simulink model "test_MCU_RTI1202_20180630"  (R2017a)
settings: Solver=FixedStepDiscrete  StartTime=0.0  StopTime=Inf  FixedStep=0.05  RelTol=1e-3
PostLoadFcn:
  | , if any(exist('dsrtsu_mdlpostloadfcn', 'file') == [2, 3, 6]), try dsrtsu_mdlpostloadfcn('Execute', bdroot); catch fprintf('Error in PostLoadFcn (dsrtsu_mdlpostloadfcn) for model "%s":\n %s\n', bdroot, lasterr); end, end,
libraries: rti1202serlib x4
settings Model: DSRTSU_INTERNAL_RTI_VER=500  DSRTSU_INTERNAL_RTI_TYPE=rti1202  RTICANMMDATA=struct('GeneralSetupData',struct('modelroot',['L:\New folder\REC_Maroje\Demo1\RTI\Demos\Model\DS1202\Model'],'generalsettings',struct('filesettings',struct('destfolder',struct('Name','RTICANMM_FILES','Check',1),'buildfolder',struct('Name','.','Check',1),'AbsDestfolder',struct('Name',['L:\New folder\REC_Maroje\Demo1\RTI\Demos\Model\DS1202\Model\RTICANMM_FILES']),'AbsBuildfolder',struct('Name',['L:\New folder\REC_Maroje\Demo1\RTI\Demos\Model\DS1202\Model']))),'options',struct('addpaths',1,'rmpaths',1,'addtrcexclusion',logical(1),'cannavigator',struct('checkmonitoring',0),'show_usrtrc',0,'use_usrtrc',0),'advanced',struct('options',ones(1,100)),'MPSetup',{{}},'modelname','demo1202_serial_4','block','demo1202_serial_4'))  DSRTSU_INTERNAL_RTIFLEXRAYCONFIG=110  DSRTSU_INTERNAL_RTIFPGA=90  ExtModeTrigMode=oneshot  ExtModeArmWhenConnect=off  ExtModeAutoUpdateStatusClock=off  Creator=dSPACE GmbH  LastModifiedBy=kiritsuPC
settings DataIOCC: LimitDataPoints=on  SaveFormat=Array  SignalLoggingSaveFormat=ModelDataLogs
settings OptimizationCC: BlockReduction=off  ConditionallyExecuteInputs=off  OptimizeBlockIOStorage=off  BufferReuse=off  GlobalBufferReuse=off  ExpressionFolding=off  ExpressionDepthLimit=2147483647  LocalBlockOutputs=off  InitFltsAndDblsToZero=on  LifeSpan=inf
settings DebuggingCC: SaveWithParameterizedLinksMsg=none  UnderspecifiedInitializationDetection=Classic  MergeDetectMultiDrivingBlocksExec=none  SignalResolutionControl=TryResolveAllWithWarning  SolverPrmCheckMsg=warning  MultiTaskDSMMsg=warning  MultiTaskCondExecSysMsg=none  MultiTaskRateTransMsg=warning  TasksWithSamePriorityMsg=none  FcnCallInpInsideContextMsg=warning  AllowSymbolicDim=off  StateNameClashWarn=warning  SFUnexpectedBacktrackingDiag=warning  SFNoUnconditionalDefaultTransitionDiag=warning  SFExecutionAtInitializationDiag=none
settings HardwareCC: ProdBitPerPointer=32  ProdBitPerSizeT=32  ProdBitPerPtrDiffT=32  ProdLargestAtomicInteger=Integer  ProdEndianess=BigEndian  ProdWordSize=32  ProdHWDeviceType=Custom Processor->Custom  TargetIntDivRoundTo=Zero  TargetEndianess=BigEndian  TargetHWDeviceType=Custom Processor->Custom
settings ModelReferenceCC: PropagateSignalLabelsOutOfModel=off
settings SFSimCC: MATLABDynamicMemAlloc=off
settings RTWCC: SystemTargetFile=rti1202.tlc  MakeCommand=make_rti  TemplateMakefile=rti1202.tmf  Description=dSPACE DS1202 Hardware Platform  RTWVerbose=off
settings STFCustomTargetCC: ParMdlRefBuildCompliant=on  GRTInterface=off  SystemTargetFile=rti1202.tlc
settings GRTTargetCC: TargetLangStandard=C89/C90 (ANSI)  CompOptLevelCompliant=off  ConcurrentExecutionCompliant=off  CombineOutputUpdateFcns=off  MatFileLogging=off  CPPClassGenCompliant=off  UseToolchainInfoCompliant=off  ExtModeMexFile=noextcomm
settings ConfigComp: CovMetricSettings=dw  CovHtmlReporting=on  CovSaveCumulativeToWorkspaceVar=on  CovSaveSingleToWorkspaceVar=on  CovExternalEMLEnable=off

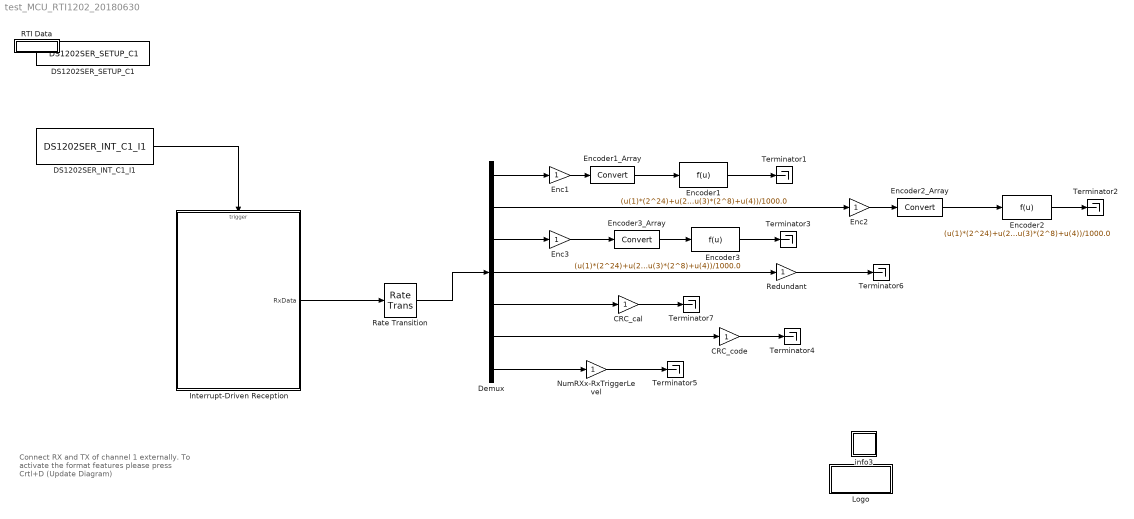
== system test_MCU_RTI1202_20180630 ==
  note: Connect RX and TX of channel 1 externally.
      | To activate the format features please
      | press Crtl+D (Update Diagram)
  CRC_cal : Gain  SaturateOnIntegerOverflow=on  OutDataTypeStr=Inherit: Same as input  ParamDataTypeStr=Inherit: Same as input
  CRC_code : Gain  SaturateOnIntegerOverflow=on  OutDataTypeStr=Inherit: Same as input  ParamDataTypeStr=Inherit: Same as input
  DS1202SER_INT_C1_I1 : rti1202serlib/DS1202SER_INT_C1_I1  Reserved1=[]  Reserved2=[]  Reserved3=[]  Reserved4=[]  DSProperties=struct('RTI',struct('IOBoardType',{{'DS1202','SER'}},'SlaveProcessor','NONE','Version',uint32(3),'BlockType',struct('isSLSource',uint8(1),'isSLSink',uint8(0),'isHWSource',uint8(0),'isHWSink',uint8(0),'isSetup',uint8(0),'isInline',uint8(1),'isNonInline',uint8(0),'isInterrupt',uint8(1),'isChannelwise',uint8(1)),'UnitType','GENSER','Identifier','SERINT','DialogType','ML','BlockSet','NONE','RelationId',struct('TH',struct('BlockId','HWINT'))))  RTIBlockInterface=struct('BlockDisplay',{{['DS1202 SER Interrupt\n Channel 1\nReceive Interrupt'],'center'}},'BlockName',struct('Token',{{'DS1202SER_INT_C','_I'}},'BlockParam',{{'ChannelNo','IntType'}}),'OutputPortsWidth',int32(1),'OutputPortsActive',1,'OutputPortsName',{{[' ']}},'IconTransparency','off','ParameterTunableNames',{{}},'InitLevel',3,'DialogFcn','guigenserserint','MaskDescription',['To make the interrupts of the UART serial interface available as trigger source.'],'FunctionCall',uint32(0),'Options',{{'SS_OPTION_FORCE_NONINLINED_FCNCALL','SS_OPTION_ASYNCHRONOUS_INTERRUPT'}})  RTIBlockParameters=struct('ThIntNo',{{'UART_EVENTS','OFF',[]}},'ThSubIntNo',{{0,'ON',[0 4]}},'ThSrcSgnName',{{['UART Ch1 RX SW FIFO interrupt'],'OFF',[]}},'TLCFileName',{{'rti_hwinterrupt','OFF',[]}},'BoardNo',{{1,'ON',[1 1]}},'ChannelNo',{{1,'ON',[1 2]}},'ChannelNumOf',{{2,'OFF',[]}},'ThBlk',{{['struct(''blkh'',''test_MCU_RTI1202_20180630/DS1202SER_INT_C1_I1'',''srcId'',''UART_EVENTS_CH1_INT0'',''srcSgnId'',''UART_EVENTS_CH1_INT0'',''intervalTmrBlockId'',[],''srcSgnName'',[''UART Ch1 RX SW FIFO interrupt''],''srcCpuId'','''',''isSrcCpu'',1,''isTargetCpu'',1,''srcOnMasterCpu'',1,''boardType'','''',''boardTypeNo'','''',''boardNo'',1,''intNo'',''UART_EVENTS'',''subIntNo'',0,''period'',0,''entryPoint'',''rti_UART_EVENTS_CH1_INT0'',''blockName'',''DS1202SER_INT_C1_I1'',''taskNameDisplayExt'','''',''taskType'',''HWINT'',''groupId'',''SERINT'',''hookFcn'',''NULL'',''isTimerTaskSrc'',0,''service'','''',''mpBlkId'','''',''taskPriorityPreConfig'',''none'',''taskPriority'',-1,''taskSortWeighting'',[],''taskSchedulingPolicy'',''FCFS'',''taskOvrPreConfig'',''none'',''taskOvrStrategy'',1,''taskOvrQueueSize'',1,''taskVisibility'',''on'',''taskGroupId'','''',''taskGroupDisplayOrder'',[],''serviceDynamicGen'',0,''disableCodeGen'',0,''boardBase'',''IOLIB_SPEC_INT_UART(1)'',''noBoardBase'','''')'],'OFF',[]}},'IntType',{{1,'ON',[1 4]}},'ReceiveIntLevelFifo',{{'13','OFF',[]}},'IntTypeMacro',{{'DSSER_TRIGGER_LEVEL_SUBINT_MASK','OFF',[]}},'FifoSizeDefault',{{64,'OFF',[]}})  RTISFcnParameters=struct('BoardNo','double','ChannelNo','double','ThIntNo','double','ThSubIntNo','double','ThBlk','struct','IntType','double','ReceiveIntLevelFifo','double','TLCFileName','char','IntTypeMacro','char')  RTIBlockParaDefault=struct('ThIntNo',1,'ThSubIntNo',0,'ThSrcSgnName',['RX SW FIFO interrupt'],'TLCFileName','rti_hwinterrupt','BoardNo',1,'ChannelNo',1,'ChannelNumOf',2,'ThBlk',['struct(''srcSgnId'', '''')'],'IntType',1,'ReceiveIntLevelFifo',1,'IntTypeMacro','DSSER_TRIGGER_LEVEL_SUBINT_MASK','FifoSizeDefault',64)
  DS1202SER_SETUP_C1 : rti1202serlib/DS1202SER_SETUP_C1  Reserved1=[]  Reserved2=[]  Reserved3=[]  Reserved4=[]  DSProperties=struct('RTI',struct('Version',uint32(2),'IOBoardType',{{'DS1202','SER'}},'SlaveProcessor','NONE','BlockType',struct('isSLSource',uint8(0),'isSLSink',uint8(0),'isHWSource',uint8(0),'isHWSink',uint8(0),'isSetup',uint8(1),'isInline',uint8(1),'isNonInline',uint8(0),'isInterrupt',uint8(0),'isChannelwise',uint8(1)),'UnitType','GENSER','Identifier','SETUP','DialogType','ML','BlockSet','NONE'))  RTIBlockInterface=struct('BlockName',struct('Token',{{'DS1202SER_SETUP_C'}},'BlockParam',{{'ChannelNo'}}),'BlockDisplay',{{['Serial Setup'],'center'}},'IconTransparency','off','ParameterTunableNames',{{}},'InitLevel',1,'DialogFcn','guigensersetup','MaskDescription',['To set the global specifications for the UART interface.'])  RTIBlockParameters=struct('ParityMode',{{1,'OFF',[1 5]}},'TransceiverMode',{{[3;1],'OFF',[]}},'QuartzFrequency',{{'160000000','OFF',[]}},'BoardNo',{{1,'ON',[1 1]}},'ChannelNo',{{1,'ON',[1 2]}},'ChannelNumOf',{{2,'OFF',[]}},'BaudRate',{{'115200','OFF',[]}},'DataBitsNumOf',{{4,'OFF',[1 4]}},'StopBitsNumOf',{{1,'OFF',[1 3]}},'ReceiveIntLevelUart',{{1,'OFF',[1 4]}},'AutoflowMode',{{0,'OFF',[]}},'FifoSize',{{'64','OFF',[]}},'ReceiveIntLevelFifo',{{0,'OFF',[]}},'FifoOverrunMode',{{1,'OFF',[]}},'FifoBlockSize',{{'0','OFF',[]}},'TermMode',{{1,'OFF',[]}},'TLCFileName',{{'rtigensersetup','OFF',[]}})  RTISFcnParameters=struct('BoardNo','double','ChannelNo','double','ChannelNumOf','double','BaudRate','double','DataBitsNumOf','double','StopBitsNumOf','double','ParityMode','double','TransceiverMode','double','ReceiveIntLevelUart','double','AutoflowMode','double','FifoSize','double','ReceiveIntLevelFifo','double','FifoBlockSize','double','TermMode','double','QuartzFrequency','double','TLCFileName','char')  RTIBlockParaDefault=struct('ParityMode',1,'TransceiverMode',[1;1],'QuartzFrequency',160000000,'BoardNo',1,'ChannelNo',1,'ChannelNumOf',2,'BaudRate',115200,'DataBitsNumOf',4,'StopBitsNumOf',1,'ReceiveIntLevelUart',4,'AutoflowMode',0,'FifoSize',64,'ReceiveIntLevelFifo',0,'FifoOverrunMode',1,'FifoBlockSize',0,'TermMode',1,'TLCFileName','rtigensersetup')
  Demux : Demux  Outputs=[4, 4, 4, 2, 1,1,2]
  Enc1 : Gain  SaturateOnIntegerOverflow=on  OutDataTypeStr=Inherit: Same as input  ParamDataTypeStr=Inherit: Same as input
  Enc2 : Gain  SaturateOnIntegerOverflow=on  OutDataTypeStr=Inherit: Same as input  ParamDataTypeStr=Inherit: Same as input
  Enc3 : Gain  SaturateOnIntegerOverflow=on  OutDataTypeStr=Inherit: Same as input  ParamDataTypeStr=Inherit: Same as input
  Encoder1 : Fcn  Expr=(u(1)*(2^24)+u(2)*(2^16)+u(3)*(2^8)+u(4))/1000.0
  "Encoder1_Array " : DataTypeConversion  SaturateOnIntegerOverflow=on  RndMeth=Zero
  Encoder2 : Fcn  Expr=(u(1)*(2^24)+u(2)*(2^16)+u(3)*(2^8)+u(4))/1000.0
  Encoder2_Array : DataTypeConversion  SaturateOnIntegerOverflow=on  RndMeth=Zero
  Encoder3 : Fcn  Expr=(u(1)*(2^24)+u(2)*(2^16)+u(3)*(2^8)+u(4))/1000.0
  "Encoder3_Array " : DataTypeConversion  SaturateOnIntegerOverflow=on  RndMeth=Zero
  Interrupt-Driven Reception : Subsystem  TreatAsAtomicUnit=on
  Logo : Subsystem  mask(dSPACE){EmptyParameter=[]}
      mask prompts: EmptyParameter "Mask Parameter 1:"
      settings: OpenFcn=;
      mask Display: image(imread('rti_mdl_dslogo.tif'));
  NumRXx-RxTriggerLevel : Gain  SaturateOnIntegerOverflow=on  OutDataTypeStr=Inherit: Same as input  ParamDataTypeStr=Inherit: Same as input
  RTI Data : Subsystem  Tag=struct('RTIDataServer',struct('RTIDataServerVs','2','RTIModelDescription','struct(''main'',''test_MCU_RTI1202_20180630'',''sub'','''',''isMp'',0)'))  LoadFcn="if exist('rtidc'), try,  rtidc('DataHostBlockClbLoad', gcbh); catch, disp(['Warning: ''LoadFcn'' for RTI Data block failed: ' lasterr]); end, end,"  mask(RTI_DATA_HOST){}
      mask help:
      | RTI Data Block.
      | This block is used by RTI to store internal model-dependent data.
      | Please keep this block on the root level of the model. Deleting this block will result in data loss.
      |
      | NEVER DELETE OR COPY THIS BLOCK!
      settings: CopyFcn="if exist('rtidc'), try,  rtidc('DataHostBlockClbCopy', gcbh); catch, disp(['Warning: ''CopyFcn'' for RTI Data block failed: ' lasterr]); end, end,"  DeleteFcn="if exist('rtidc'), try,  rtidc('DataHostBlockClbDelete', gcbh); catch, disp(['Warning: ''DeleteFcn'' for RTI Data block failed: ' lasterr]); end, end,"  ModelCloseFcn="if exist('rtidc'), try,  rtidc('DataHostBlockClbModelClose', gcbh); catch, disp(['Warning: ''ModelCloseFcn'' for RTI Data block failed: ' lasterr]); end, end,"  PreSaveFcn="if exist('rtidc'), try,  rtidc('DataHostBlockClbPreSave', gcbh); catch, disp(['Warning: ''PreSaveFcn'' for RTI Data block failed: ' lasterr]); end, end,"  PostSaveFcn="if exist('rtidc'), try,  rtidc('DataHostBlockClbPostSave', gcbh); catch, disp(['Warning: ''PostSaveFcn'' for RTI Data block failed: ' lasterr]); end, end,"  NameChangeFcn="if exist('rtidc'), try,  rtidc('DataHostBlockClbNameChange', gcbh); catch, disp(['Warning: ''NameChangeFcn'' for RTI Data block failed: ' lasterr]); end, end,"
      mask Help:
      | RTI Data Block.
      | This block is used by RTI to store internal model-dependent data.
      | Please keep this block on the root level of the model. Deleting this block will result in data loss.
      | 
      | NEVER DELETE OR COPY THIS BLOCK!
      mask Display:
      | text(0.5, 0.5, 'RTI Data', 'HorizontalAlignment', 'center');
      | plot([1 0]);
  Rate Transition : RateTransition  Integrity=off
  Redundant : Gain  SaturateOnIntegerOverflow=on  OutDataTypeStr=Inherit: Same as input  ParamDataTypeStr=Inherit: Same as input
  Terminator{1..7} (7 alike) : Terminator
  info3 : Subsystem
      settings: OpenFcn=web(fullfile(dspaceroot, 'demos', rtitype('processorboard'), 'rti', 'demo1xxx_serial_4.html'), '-browser');
      mask Display: disp('?')
  wires:
  DS1202SER_INT_C1_I1/1 -> Interrupt-Driven Reception/Trigger
  Interrupt-Driven Reception/1(RxData) -> Rate Transition/1
  Rate Transition/1 -> Demux/1
  NumRXx-RxTriggerLevel/1 -> Terminator5/1
  CRC_code/1 -> Terminator4/1
  Encoder3/1 -> Terminator3/1
  Encoder2/1 -> Terminator2/1
  Encoder1/1 -> Terminator1/1
  Redundant/1 -> Terminator6/1
  Demux/1 -> Enc1/1
  "Encoder1_Array "/1 -> Encoder1/1
  Encoder2_Array/1 -> Encoder2/1
  Demux/2 -> Enc2/1
  Demux/3 -> Enc3/1
  "Encoder3_Array "/1 -> Encoder3/1
  Enc1/1 -> "Encoder1_Array "/1
  Enc2/1 -> Encoder2_Array/1
  Enc3/1 -> "Encoder3_Array "/1
  Demux/4 -> Redundant/1
  Demux/7 -> NumRXx-RxTriggerLevel/1
  Demux/6 -> CRC_code/1
  CRC_cal/1 -> Terminator7/1
  Demux/5 -> CRC_cal/1

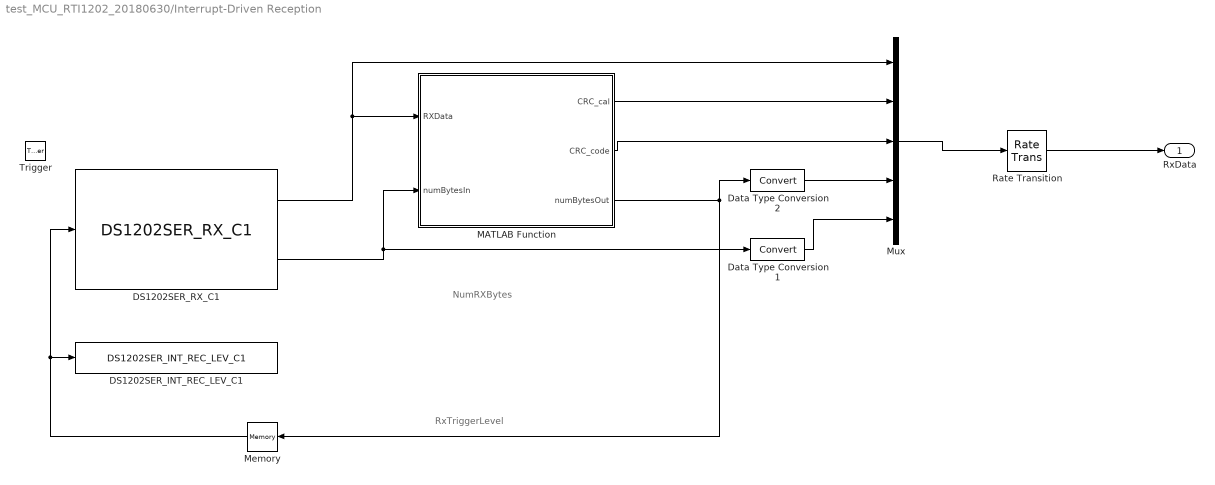
== system test_MCU_RTI1202_20180630/Interrupt-Driven Reception ==
  note: NumRXBytes
  note: RxTriggerLevel
  Trigger : TriggerPort  TriggerType=function-call  VariantControl=Variant
  DS1202SER_INT_REC_LEV_C1 : rti1202serlib/DS1202SER_INT_REC_LEV_C1  Reserved1=[]  Reserved2=[]  Reserved3=[]  Reserved4=[]  DSProperties=struct('RTI',struct('IOBoardType',{{'DS1202','SER'}},'SlaveProcessor','NONE','Version',uint32(1),'BlockType',struct('isSLSource',uint8(1),'isSLSink',uint8(0),'isHWSource',uint8(0),'isHWSink',uint8(0),'isSetup',uint8(0),'isInline',uint8(1),'isNonInline',uint8(0),'isInterrupt',uint8(0),'isChannelwise',uint8(1)),'UnitType','GENSER','Identifier','INTLEV','DialogType','ML','BlockSet','NONE'))  RTIBlockInterface=struct('BlockName',struct('Token',{{'DS1202SER_INT_REC_LEV_C'}},'BlockParam',{{'ChannelNo'}}),'InputPortsWidth',int32(1),'InputPortsActive',1,'InputPortsDataType',{{'SS_UINT32'}},'InputPortsName',{{['Receive SW FIFO Threshold']}},'IWork',{{{'',uint32(1)}}},'BlockDisplay',{{['Serial Interrupt \nReceive SW FIFO Threshold'],'center'}},'IconTransparency','off','ParameterTunableNames',{{}},'InitLevel',1,'DialogFcn','guigenserintlev','MaskDescription',['To read the contents of the UART status register.'])  RTIBlockParameters=struct('BoardNo',{{1,'ON',[1 1]}},'ChannelNo',{{1,'ON',[1 2]}},'ChannelNumOf',{{2,'OFF',[]}},'ReceiveIntLevelFifo',{{0,'OFF',[]}},'SetupFifoBlockSize',{{0,'OFF',[]}},'SetupBaudRate',{{115200,'OFF',[]}},'SetupDataBitsNumOf',{{8,'OFF',[]}},'SetupStopBitsNumOf',{{1,'OFF',[]}},'SetupParityMode',{{'NO_PARITY','OFF',[]}},'SetupReceiveIntLevelUart',{{1,'OFF',[]}},'SetupTransceiverMode',{{'RS485','OFF',[]}},'SetupAutoflowMode',{{'DISABLE','OFF',[]}},'TLCFileName',{{'rtigenserintlev','OFF',[]}})  RTISFcnParameters=struct('BoardNo','double','ChannelNo','double','ChannelNumOf','double','ReceiveIntLevelFifo','double','SetupFifoBlockSize','double','SetupBaudRate','double','SetupDataBitsNumOf','double','SetupStopBitsNumOf','double','SetupParityMode','char','SetupReceiveIntLevelUart','double','SetupTransceiverMode','char','SetupAutoflowMode','char','TLCFileName','char')  RTIBlockParaDefault=struct('BoardNo',1,'ChannelNo',1,'ChannelNumOf',2,'ReceiveIntLevelFifo',0,'SetupFifoBlockSize',0,'SetupBaudRate',0,'SetupDataBitsNumOf',0,'SetupStopBitsNumOf',0,'SetupParityMode','0','SetupReceiveIntLevelUart',0,'SetupTransceiverMode','0','SetupAutoflowMode','0','TLCFileName','rtigenserintlev')
  DS1202SER_RX_C1 : rti1202serlib/DS1202SER_RX_C1  Reserved1=[]  Reserved2=[]  Reserved3=[]  Reserved4=[]  DSProperties=struct('RTI',struct('IOBoardType',{{'DS1202','SER'}},'SlaveProcessor','NONE','Version',uint32(1),'BlockType',struct('isSLSource',uint8(1),'isSLSink',uint8(1),'isHWSource',uint8(0),'isHWSink',uint8(1),'isSetup',uint8(0),'isInline',uint8(1),'isNonInline',uint8(0),'isInterrupt',uint8(0),'isChannelwise',uint8(1)),'UnitType','GENSER','Identifier','RECEIVE','DialogType','ML','BlockSet','NONE'))  RTIBlockInterface=struct('BlockName',struct('Token',{{'DS1202SER_RX_C'}},'BlockParam',{{'ChannelNo'}}),'InputPortsWidth',int32(1),'InputPortsActive',1,'InputPortsDataType',{{'SS_UINT32'}},'InputPortsName',{{'NumBytes'}},'OutputPortsWidth',int32([14 1 1]),'OutputPortsActive',[1 1 0],'OutputPortsDataType',{{'SS_UINT8','SS_UINT32','SS_INT32'}},'OutputPortsName',{{'RXBytes','NumRXBytes','Status'}},'BlockDisplay',{{['Serial Receive'],'center'}},'IconTransparency','on','ParameterTunableNames',{{'BytesRefNumOf'}},'InitLevel',2,'DialogFcn','guigenserreceive','MaskDescription',['To read data from the UART SW FIFO.'])  RTIBlockParameters=struct('BoardNo',{{1,'ON',[1 1]}},'ChannelNo',{{1,'ON',[1 2]}},'ChannelNumOf',{{2,'OFF',[]}},'ReceptionDataMode',{{1,'OFF',[]}},'ParamTunableMode',{{1,'OFF',[]}},'BytesRefNumOfT',{{'1','OFF',[1 inf]}},'BytesRefNumOfNT',{{'1','OFF',[1 inf]}},'BytesRefNumOfMax',{{'14','OFF',[1 inf]}},'BytesRefNumOfMode',{{0,'OFF',[]}},'BytesActNumOfMode',{{1,'OFF',[]}},'ReceptionStatusMode',{{0,'OFF',[]}},'FifoSizeDefault',{{64,'OFF',[]}},'TLCFileName',{{'rtigenserreceive','OFF',[]}})  RTISFcnParameters=struct('BoardNo','double','ChannelNo','double','ChannelNumOf','double','ReceptionDataMode','double','ParamTunableMode','double','BytesRefNumOfT','double','BytesRefNumOfNT','double','BytesRefNumOfMax','double','BytesRefNumOfMode','double','BytesActNumOfMode','double','ReceptionStatusMode','double','TLCFileName','char')  RTIBlockParaDefault=struct('BoardNo',1,'ChannelNo',1,'ChannelNumOf',2,'ReceptionDataMode',1,'ParamTunableMode',1,'BytesRefNumOfT',1,'BytesRefNumOfNT',1,'BytesRefNumOfMax',1,'BytesRefNumOfMode',0,'BytesActNumOfMode',1,'ReceptionStatusMode',1,'FifoSizeDefault',64,'TLCFileName','rtigenserreceive')
  Data Type Conversion1 : DataTypeConversion  SaturateOnIntegerOverflow=on  RndMeth=Zero
  Data Type Conversion2 : DataTypeConversion  SaturateOnIntegerOverflow=on  RndMeth=Zero
  MATLAB Function : MATLAB Function  TreatAsAtomicUnit=on
  Memory : Memory  X0=1  InheritSampleTime=on
  Mux : Mux  Inputs=5
  Rate Transition : RateTransition  Integrity=off
  RxData : Outport
  wires:
  DS1202SER_RX_C1/2 -> MATLAB Function/2(numBytesIn), Data Type Conversion1/1
  Mux/1 -> Rate Transition/1
  Memory/1 -> DS1202SER_RX_C1/1, DS1202SER_INT_REC_LEV_C1/1
  DS1202SER_RX_C1/1 -> Mux/1, MATLAB Function/1(RXData)
  MATLAB Function/3(numBytesOut) -> Memory/1, Data Type Conversion2/1
  Rate Transition/1 -> RxData/1
  Data Type Conversion1/1 -> Mux/5
  Data Type Conversion2/1 -> Mux/4
  MATLAB Function/2(CRC_code) -> Mux/3
  MATLAB Function/1(CRC_cal) -> Mux/2

== system test_MCU_RTI1202_20180630/Logo ==
  note: $Revision: 2.4 $
  note: $Date: 2012/07/16 15:49:27MESZ $
  note: $RCSfile: demo1401_serial_4.mdl $

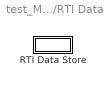
== system test_MCU_RTI1202_20180630/RTI Data ==
  RTI Data Store : Subsystem  Tag="struct('private',struct('version',struct('dsVer',uint32(2),'dsVerCreation',uint32(2),'RTI',struct('ver','7.8','type','RTI1202')),'access',struct('type','Model','isPerm',1,'created',['30-Jun-2018 13:52:50'],'modified',['01-Jul-2018 13:00:20'],'location','')),'public',struct('main',struct('data',[]),'sub',struct('name',{{'test_MCU_RTI1202_20180630'}},'data',{{struct('TH',struct('thTaskInfo',struct('taskType',{'TIMER','HWINT','TMRINT','SWINT','GLINT'},'tasksNumOf',{1,1,0,0,0},'srcIds',{{'TIMERA'},{'UART_EVENTS_CH1_INT0'},{},{},{}},'taskNames',{{['Timer Task 1']},{'DS1202SER_INT_C1_I1'},{},{},{}})),'th_tc',struct('dataType',{'TASK','TASK'},'taskGroupId',{'',''},'taskGroupList',{{},{}},'taskSchedulingPolicy',{'FCFS','FCFS'},'taskType',{'TIMER','HWINT'},'blkh',{-1,'test_MCU_RTI1202_20180630/DS1202SER_INT_C1_I1'},'srcId',{'TIMERA','UART_EVENTS_CH1_INT0'},'srcSgnName',{['Timer A interrupt'],['UART Ch1 RX SW FIFO interrupt']},'srcCpuName',{'',''},'taskName',{['Timer Task 1  [0.05] s'],'DS1202SER_INT_C1_I1'},'taskNameDisplayExt',{'',''},'smplTime',{0.05,0},'smplTimeOffs',{0,0},'hasFixedPriority',{0,0},'priority',{1,2},'hasFixedOvc',{0,0},'ovcType',{1,1},'ovcMax',{1,1}),'tc_th',struct('dataType',{'TASK','TASK'},'taskGroupId',{'',''},'taskGroupList',{{},{}},'taskSchedulingPolicy',{'FCFS','FCFS'},'taskType',{'TIMER','HWINT'},'blkh',{-1,'test_MCU_RTI1202_20180630/DS1202SER_INT_C1_I1'},'srcId',{'TIMERA','UART_EVENTS_CH1_INT0'},'srcSgnName',{['Timer A interrupt'],['UART Ch1 RX SW FIFO interrupt']},'srcCpuName',{'',''},'taskName',{['Timer Task 1  [0.05] s'],'DS1202SER_INT_C1_I1'},'taskNameDisplayExt',{'',''},'smplTime',{0.05,0},'smplTimeOffs',{0,0},'hasFixedPriority',{0,0},'priority',{1,2},'hasFixedOvc',{0,0},'ovcType',{1,1},'ovcMax',{1,1}))}})))"  mask(RTI_DATA_STORE){}
      mask help:
      | RTI Data Store Block. This block is used by RTI to store internal model dependent data. Deleting this block will result in data loss.
      |
      | NEVER DELETE, COPY, OR MODIFY THIS BLOCK!
      mask Help:
      | RTI Data Store Block. This block is used by RTI to store internal model dependent data. Deleting this block will result in data loss.
      | 
      | NEVER DELETE, COPY, OR MODIFY THIS BLOCK!
      mask Display: text(0.5, 0.5, ' ', 'HorizontalAlignment', 'center');

== system test_MCU_RTI1202_20180630/info3 ==

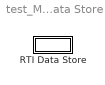
== system test_MCU_RTI1202_20180630/RTI Data/RTI Data Store ==
  RTI Data Store : Subsystem  mask(RTI_DATA_STORE){}
      mask help:
      | RTI Data Store Block. This block is used by RTI to store internal model dependent data. Deleting this block will result in data loss.
      |
      | NEVER DELETE, COPY, OR MODIFY THIS BLOCK!
      mask Help:
      | RTI Data Store Block. This block is used by RTI to store internal model dependent data. Deleting this block will result in data loss.
      | 
      | NEVER DELETE, COPY, OR MODIFY THIS BLOCK!
      mask Display: text(0.5, 0.5, ' ', 'HorizontalAlignment', 'center');

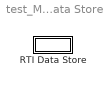
== system test_MCU_RTI1202_20180630/RTI Data/RTI Data Store/RTI Data Store ==
  RTI Data Store : Subsystem  mask(RTI_DATA_STORE){}
      mask help:
      | RTI Data Store Block. This block is used by RTI to store internal model dependent data. Deleting this block will result in data loss.
      |
      | NEVER DELETE, COPY, OR MODIFY THIS BLOCK!
      mask Help:
      | RTI Data Store Block. This block is used by RTI to store internal model dependent data. Deleting this block will result in data loss.
      | 
      | NEVER DELETE, COPY, OR MODIFY THIS BLOCK!
      mask Display: text(0.5, 0.5, ' ', 'HorizontalAlignment', 'center');

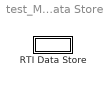
== system test_MCU_RTI1202_20180630/RTI Data/RTI Data Store/RTI Data Store/RTI Data Store ==
  RTI Data Store : Subsystem  mask(RTI_DATA_STORE){}
      mask help:
      | RTI Data Store Block. This block is used by RTI to store internal model dependent data. Deleting this block will result in data loss.
      |
      | NEVER DELETE, COPY, OR MODIFY THIS BLOCK!
      mask Help:
      | RTI Data Store Block. This block is used by RTI to store internal model dependent data. Deleting this block will result in data loss.
      | 
      | NEVER DELETE, COPY, OR MODIFY THIS BLOCK!
      mask Display: text(0.5, 0.5, ' ', 'HorizontalAlignment', 'center');

== system test_MCU_RTI1202_20180630/RTI Data/RTI Data Store/RTI Data Store/RTI Data Store/RTI Data Store ==

== matlab function test_MCU_RTI1202_20180630/Interrupt-Driven Reception/MATLAB Function ==
  data: CRC_cal output; CRC_code output; numBytesOut output; RXData input; numBytesIn input
function [CRC_cal, CRC_code, numBytesOut] = Calculate(RXData, numBytesIn)

crc_table = uint8(zeros(1, 256));
generator = uint8(29); % hex2dec('1D')
last_bit = uint8(128); % hex2dec('80')
for divident = 1:256
    currentByte = uint8(divident-1);
    % calculate the CRC-8 value for current byte
    for bit = 1:8
        if (bitand(currentByte, last_bit))
            currentByte = bitshift(currentByte, 1, 'uint8'); % <<= 1
            currentByte = bitxor(currentByte, generator, 'uint8');
        else 
            currentByte = bitshift(currentByte, 1, 'uint8'); % <<= 1
        end
    end
    % store CRC value in lookup table
    crc_table(1, divident) = currentByte;
end
crc_table(1, 1) = 1;

% Calculate CRC code
CRC_cal = uint8(171); % 0xAB

for i=1:12
    idata = uint8(RXData(i + numBytesIn - 13));   % 0~255
    index = bitxor(CRC_cal, idata, 'uint8');      % 0~255
    CRC_cal = uint8(crc_table(1, 1+index));
%     fprintf('id=%d, CRC_cal=%d \n', index, CRC_cal);
end


CRC_code = uint8(RXData(numBytesIn));
    
if CRC_cal == CRC_code
    numBytesOut = uint32(13);
else 
    numBytesOut = uint32(14);
end
